simulink model "simulation_w_switch"  (Simulink 10.0)
settings: Solver=VariableStepAuto  StartTime=0.0  StopTime=tTot  MaxStep=1e-4  RelTol=1e-3
PreLoadFcn:
  | syst_init
values from neighbouring files (symbols this model uses):
  D = diag(Ir.^-1)    [syst_init.m]
  DGU = stateDyn(DGU,6)    [syst_init.m]
  Il_bar1 = 5/3    (= 1.66666666667)    [syst_init.m]
  Il_bar2 = 6/3    (= 2)    [syst_init.m]
  Il_bar3 = 7/3    (= 2.33333333333)    [syst_init.m]
  Il_bar4 = 6.5/3    (= 2.16666666667)    [syst_init.m]
  Il_bar5 = 8/3    (= 2.66666666667)    [syst_init.m]
  Il_bar6 = 7.5/3    (= 2.5)    [syst_init.m]
  L_first = Bc_first*Wcomm_first*(Bc_first')    [syst_init.m]
  L_full = Bc_full*Wcomm_full*(Bc_full')    [syst_init.m]
  L_unp = Bc_unp*Wcomm_unp*(Bc_unp')    [syst_init.m]
  N = 6    [syst_init.m]
  Pl_bar1 = 100/3    (= 33.3333333333)    [syst_init.m]
  Pl_bar2 = 120/3    (= 40)    [syst_init.m]
  Pl_bar3 = 105/3    (= 35)    [syst_init.m]
  Pl_bar4 = 95/3    (= 31.6666666667)    [syst_init.m]
  Pl_bar5 = 110/3    (= 36.6666666667)    [syst_init.m]
  Pl_bar6 = 105/3    (= 35)    [syst_init.m]
  T_zie_change = 17    [syst_init.m]
  T_zip_change = 6    [syst_init.m]
  Tc = 1.5    [syst_init.m]
  Tcommfail = tTot-3    (= 26)    [syst_init.m]
  Tplg = 10    [syst_init.m]
  Tunp = 22    [syst_init.m]
  Vref1 = 47    [syst_init.m]
  Vref2 = 48    [syst_init.m]
  Vref3 = 45    [syst_init.m]
  Vref4 = 50    [syst_init.m]
  Vref5 = 46    [syst_init.m]
  Vref6 = 49    [syst_init.m]
  Vs = 80    [syst_init.m]
  Yl_bar1 = 1/10/3    (= 0.0333333333333)    [syst_init.m]
  Yl_bar2 = 1/9/3    (= 0.037037037037)    [syst_init.m]
  Yl_bar3 = 1/11/3    (= 0.030303030303)    [syst_init.m]
  Yl_bar4 = 1/11/3    (= 0.030303030303)    [syst_init.m]
  Yl_bar5 = 1/10/3    (= 0.0333333333333)    [syst_init.m]
  Yl_bar6 = 1/10.5/3    (= 0.031746031746)    [syst_init.m]
undefined symbols (not defined in the file or in its folder): L
libraries: powerlib x135, powerlib_meascontrol x6
(part 2 of 2)

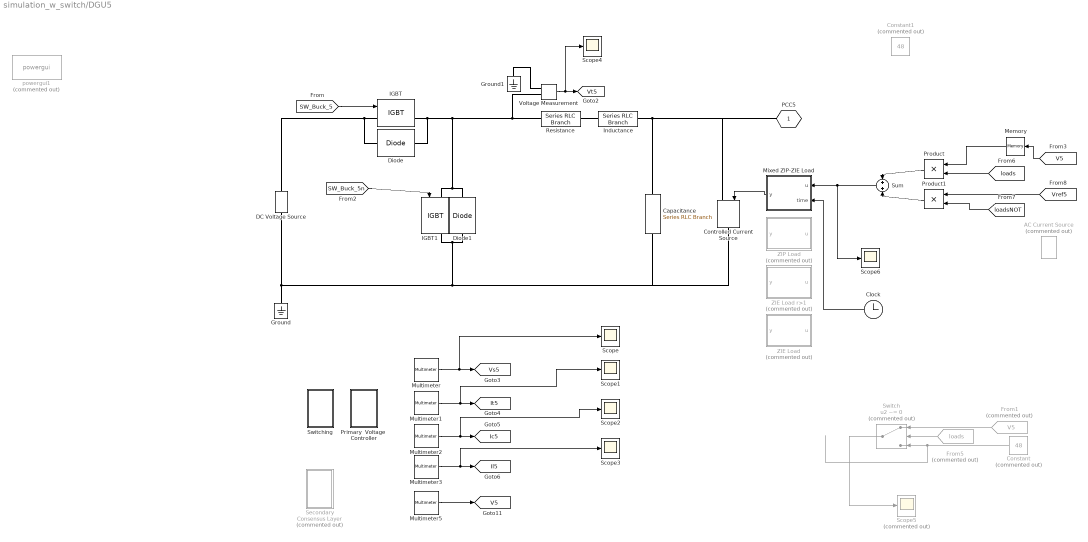
== system simulation_w_switch/DGU5 ==
  AC Current Source : powerlib/Electrical Sources/AC Current Source  Commented=on  Amplitude=18  Phase=90  Frequency=0  SampleTime=0  Measurements=Current
      settings: SourceProductName=Simscape Electrical  SourceProductBaseCode=PS
  Capacitance : powerlib/Elements/Series RLC Branch  LConnTagsString=__new0  RConnTagsString=__new0  BranchType=C  Resistance=1  Inductance=1.8e-3  SetiL0=off  InitialCurrent=0  Capacitance=DGU(5).Ct  Setx0=on  InitialVoltage=48  Measurements=Branch voltage and current
      settings: SourceProductName=Simscape Electrical
  Clock : Clock
  Constant : Constant  Commented=on  Value=48
  Constant1 : Constant  Commented=on  Value=48
  Controlled Current Source : powerlib/Electrical Sources/Controlled Current Source  Initialize=on  Source_Type=DC  Amplitude=Il_bar5  Phase=0  Frequency=0  Measurements=Current
      settings: SourceProductName=Simscape Electrical
  DC Voltage Source : powerlib/Electrical Sources/DC Voltage Source  Amplitude=Vs  Measurements=Voltage
      settings: SourceProductName=Simscape Electrical
  Diode : powerlib/Power Electronics/Diode  Ron=0.001  Lon=0  Vf=0.8  IC=0  UseSnubber=0  Rs=500  Cs=250e-9  Measurements=off
      settings: SourceProductName=Simscape Electrical
  Diode1 : powerlib/Power Electronics/Diode  Ron=0.001  Lon=0  Vf=0.8  IC=0  UseSnubber=0  Rs=500  Cs=250e-9  Measurements=off
      settings: SourceProductName=Simscape Electrical
  From1 : From  Commented=on  GotoTag=V5  TagVisibility=global
  From5 : From  Commented=on  GotoTag=loads  TagVisibility=global
  Ground : powerlib/Elements/Ground  LConnTagsString=a
      settings: SourceProductName=Simscape Electrical
  Ground1 : powerlib/Elements/Ground  LConnTagsString=a
      settings: SourceProductName=Simscape Electrical
  IGBT : powerlib/Power Electronics/IGBT  Ron=0.001  Lon=0  Vf=1  Tf=1e-6  Tt=2e-6  IC=0  Rs=1e5  Cs=inf  Measurements=on
      settings: SourceProductName=Simscape Electrical
  IGBT1 : powerlib/Power Electronics/IGBT  Ron=0.001  Lon=0  Vf=1  Tf=1e-6  Tt=2e-6  IC=0  Rs=1e5  Cs=inf  Measurements=on
      settings: SourceProductName=Simscape Electrical
  Inductance : powerlib/Elements/Series RLC Branch  LConnTagsString=__new0  RConnTagsString=__new0  BranchType=L  Resistance=1  Inductance=DGU(5).Lt  SetiL0=on  InitialCurrent=Il_bar5  Capacitance=1e-6  Setx0=off  InitialVoltage=0  Measurements=None
      settings: SourceProductName=Simscape Electrical
  Memory : Memory
  Mixed ZIP-ZIE Load : MATLAB Function  TreatAsAtomicUnit=on
  Multimeter : powerlib/Measurements/Multimeter  PhasorSimulation=off  OutputType=Complex  sel=11  L=30  Gain=1  yselected={'Usrc: DGU5/DC Voltage Source'};  PSBOutputType=1  PSBequivalent=0  AxesSetting=[0,0.1,-100,100]  Display=0  SavedBlockNames=-11
      settings: SourceProductName=Simscape Electrical
  Multimeter1 : powerlib/Measurements/Multimeter  PhasorSimulation=off  OutputType=Complex  sel=22  L=30  Gain=1  yselected={'Ib: DGU5/Resistance'};  PSBOutputType=1  PSBequivalent=0  AxesSetting=[0,0.1,-100,100]  Display=0  SavedBlockNames=-11
      settings: SourceProductName=Simscape Electrical
  Multimeter2 : powerlib/Measurements/Multimeter  PhasorSimulation=off  OutputType=Complex  sel=21  L=30  Gain=1  yselected={'Ib: DGU5/Capacitance'};  PSBOutputType=1  PSBequivalent=0  AxesSetting=[0,0.1,-100,100]  Display=0  SavedBlockNames=-11
      settings: SourceProductName=Simscape Electrical
  Multimeter3 : powerlib/Measurements/Multimeter  PhasorSimulation=off  OutputType=Complex  sel=29  L=30  Gain=1  yselected={'Isrc: DGU5/Controlled Current Source'};  PSBOutputType=1  PSBequivalent=0  AxesSetting=[0,0.1,-100,100]  Display=0  SavedBlockNames=-11
      settings: SourceProductName=Simscape Electrical
  Multimeter5 : powerlib/Measurements/Multimeter  PhasorSimulation=off  OutputType=Complex  sel=5  L=30  Gain=1  yselected={'Ub: DGU5/Capacitance'};  PSBOutputType=1  PSBequivalent=0  AxesSetting=[0,0.1,-100,100]  Display=0  SavedBlockNames=-11
      settings: SourceProductName=Simscape Electrical
  Primary  Voltage  Controller : Subsystem
  Product : Product
  Product1 : Product
  Resistance : powerlib/Elements/Series RLC Branch  LConnTagsString=__new0  RConnTagsString=__new0  BranchType=R  Resistance=DGU(5).Rt  Inductance=1e-3  SetiL0=off  InitialCurrent=0  Capacitance=1e-6  Setx0=off  InitialVoltage=0  Measurements=Branch current
      settings: SourceProductName=Simscape Electrical
  Scope{,1..4,6} (6 alike) : Scope
  Scope5 : Scope  Commented=on
  Secondary Consensus Layer : Subsystem  Commented=on
  Sum : Sum  Inputs=+|+
  Switch : Switch  Commented=on  Criteria=u2 ~= 0  Threshold=0.1  ZeroCross=off
  Switching : Subsystem
  Voltage Measurement : powerlib/Measurements/Voltage Measurement  PhasorSimulation=off  OutputType=Complex  PSBequivalent=0
      settings: SourceProductName=Simscape Electrical
  ZIE Load : MATLAB Function  Commented=on  TreatAsAtomicUnit=on
  ZIE Load r>1 : MATLAB Function  Commented=on  TreatAsAtomicUnit=on
  ZIP Load : MATLAB Function  Commented=on  TreatAsAtomicUnit=on
  powergui1 : powerlib/powergui  Priority=1  Commented=on  SimulationMode=Continuous  SampleTime=50e-6  frequency=60  Iterations=50  frequencyindice=60  Pbase=100e6  ErrMax=1e-4  UnitsV=kV  UnitsW=MW  buscounter=0  FunctionMessages=off  echomessages=off  EnableUseOfTLC=off  CurrentSourceSwitches=off  DisableSnubberDevices=off  DisableRonSwitches=off  DisableVfSwitches=off  DisplayEquations=off  AutomaticDiscreteSolvers=off  SolverType=Tustin/Backward Euler (TBE)  Interpol=off  ExternalGateDelay=off  methode=off  Ts=100  x0status=blocks  SPID=on  SwTol=0  HookPort=off  NonlinearTolerance=1e-4  nMaxIteration=100  ContinueOnMaxIteration=off  RestoreLinks=warning  ResistiveCurrentMeasurement=off  Frange=[0:2:500]  Ylog=off  Xlog=on  ShowGrid=off  save=off  variable=ZData  structure=0  ZoomFFT=off  StartTime=0.0  cycles=1  DisplayStyle=1  fundamental=60  FreqAxis=off  MaxFrequency=1000  frequencyindicesteady=1  RmsSteady=1  display=off
      settings: SourceProductName=Simscape Electrical
  PCC5 : PMIOPort  Tag=PMCPort  Side=Left
  tag scope: Ic5=global, Il5=global, It5=global, V5=global, Vs5=global, Vt5=global
  wires:
  Multimeter/1 -> Scope/1, [Vs5]
  Multimeter2/1 -> Scope2/1, [Ic5]
  Voltage Measurement/1 -> Scope4/1, [Vt5]
  Multimeter1/1 -> Scope1/1, [It5]
  [SW_Buck_5n] -> IGBT1/1
  Multimeter3/1 -> Scope3/1, [Il5]
  [SW_Buck_5] -> IGBT/1
  Multimeter5/1 -> [V5]
  Mixed ZIP-ZIE Load/1(y) -> Controlled Current Source/1
  From5/1 -> Switch/2
  From1/1 -> Switch/1
  Constant/1 -> Switch/3
  Switch/1 -> Scope5/1
  [Vref5] -> Product1/1
  Product1/1 -> Sum/2
  Sum/1 -> Mixed ZIP-ZIE Load/1(u), Scope6/1
  [loadsNOT] -> Product1/2
  [loads] -> Product/2
  Memory/1 -> Product/1
  Product/1 -> Sum/1
  [V5] -> Memory/1
  Clock/1 -> Mixed ZIP-ZIE Load/2(time)
  connections:
  Ground1/LConn1 -- Voltage Measurement/LConn2
  IGBT1/RConn1 -- Controlled Current Source/RConn1 -- Capacitance/RConn1 -- Ground/LConn1 -- DC Voltage Source/LConn1 -- Diode1/LConn1
  Capacitance/LConn1 -- Controlled Current Source/LConn1 -- PCC5/RConn1 -- Inductance/RConn1
  IGBT/LConn1 -- Diode/RConn1 -- DC Voltage Source/RConn1
  Resistance/RConn1 -- Inductance/LConn1
  IGBT/RConn1 -- Resistance/LConn1 -- Voltage Measurement/LConn1 -- Diode1/RConn1 -- IGBT1/LConn1 -- Diode/LConn1

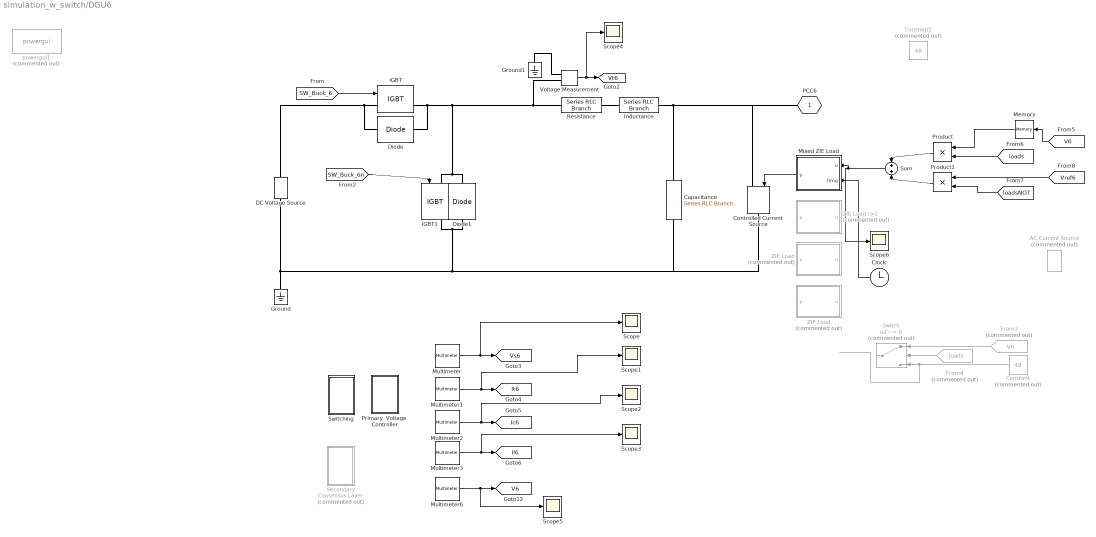
== system simulation_w_switch/DGU6 ==
  AC Current Source : powerlib/Electrical Sources/AC Current Source  Commented=on  Amplitude=16  Phase=90  Frequency=0  SampleTime=0  Measurements=Current
      settings: SourceProductName=Simscape Electrical  SourceProductBaseCode=PS
  Capacitance : powerlib/Elements/Series RLC Branch  LConnTagsString=__new0  RConnTagsString=__new0  BranchType=C  Resistance=1  Inductance=1.8e-3  SetiL0=off  InitialCurrent=0  Capacitance=DGU(6).Ct  Setx0=on  InitialVoltage=48  Measurements=Branch voltage and current
      settings: SourceProductName=Simscape Electrical
  Clock : Clock
  Constant : Constant  Commented=on  Value=48
  Constant1 : Constant  Commented=on  Value=48
  Controlled Current Source : powerlib/Electrical Sources/Controlled Current Source  Initialize=off  Source_Type=DC  Amplitude=Il_bar6  Phase=0  Frequency=0  Measurements=Current
      settings: SourceProductName=Simscape Electrical
  DC Voltage Source : powerlib/Electrical Sources/DC Voltage Source  Amplitude=Vs  Measurements=Voltage
      settings: SourceProductName=Simscape Electrical
  Diode : powerlib/Power Electronics/Diode  Ron=0.001  Lon=0  Vf=0.8  IC=0  UseSnubber=0  Rs=500  Cs=250e-9  Measurements=off
      settings: SourceProductName=Simscape Electrical
  Diode1 : powerlib/Power Electronics/Diode  Ron=0.001  Lon=0  Vf=0.8  IC=0  UseSnubber=0  Rs=500  Cs=250e-9  Measurements=off
      settings: SourceProductName=Simscape Electrical
  From3 : From  Commented=on  GotoTag=V6  TagVisibility=global
  From4 : From  Commented=on  GotoTag=loads  TagVisibility=global
  Ground : powerlib/Elements/Ground  LConnTagsString=a
      settings: SourceProductName=Simscape Electrical
  Ground1 : powerlib/Elements/Ground  LConnTagsString=a
      settings: SourceProductName=Simscape Electrical
  IGBT : powerlib/Power Electronics/IGBT  Ron=0.001  Lon=0  Vf=1  Tf=1e-6  Tt=2e-6  IC=0  Rs=1e5  Cs=inf  Measurements=on
      settings: SourceProductName=Simscape Electrical
  IGBT1 : powerlib/Power Electronics/IGBT  Ron=0.001  Lon=0  Vf=1  Tf=1e-6  Tt=2e-6  IC=0  Rs=1e5  Cs=inf  Measurements=on
      settings: SourceProductName=Simscape Electrical
  Inductance : powerlib/Elements/Series RLC Branch  LConnTagsString=__new0  RConnTagsString=__new0  BranchType=L  Resistance=1  Inductance=DGU(6).Lt  SetiL0=on  InitialCurrent=Il_bar6  Capacitance=1e-6  Setx0=off  InitialVoltage=0  Measurements=None
      settings: SourceProductName=Simscape Electrical
  Memory : Memory
  Mixed ZIE Load : MATLAB Function  TreatAsAtomicUnit=on
  Multimeter : powerlib/Measurements/Multimeter  PhasorSimulation=off  OutputType=Complex  sel=12  L=30  Gain=1  yselected={'Usrc: DGU6/DC Voltage Source'};  PSBOutputType=1  PSBequivalent=0  AxesSetting=[0,0.1,-100,100]  Display=0  SavedBlockNames=-11
      settings: SourceProductName=Simscape Electrical
  Multimeter1 : powerlib/Measurements/Multimeter  PhasorSimulation=off  OutputType=Complex  sel=24  L=30  Gain=1  yselected={'Ib: DGU6/Resistance'};  PSBOutputType=1  PSBequivalent=0  AxesSetting=[0,0.1,-100,100]  Display=0  SavedBlockNames=-11
      settings: SourceProductName=Simscape Electrical
  Multimeter2 : powerlib/Measurements/Multimeter  PhasorSimulation=off  OutputType=Complex  sel=23  L=30  Gain=1  yselected={'Ib: DGU6/Capacitance'};  PSBOutputType=1  PSBequivalent=0  AxesSetting=[0,0.1,-100,100]  Display=0  SavedBlockNames=-11
      settings: SourceProductName=Simscape Electrical
  Multimeter3 : powerlib/Measurements/Multimeter  PhasorSimulation=off  OutputType=Complex  sel=30  L=30  Gain=1  yselected={'Isrc: DGU6/Controlled Current Source'};  PSBOutputType=1  PSBequivalent=0  AxesSetting=[0,0.1,-100,100]  Display=0  SavedBlockNames=-11
      settings: SourceProductName=Simscape Electrical
  Multimeter6 : powerlib/Measurements/Multimeter  PhasorSimulation=off  OutputType=Complex  sel=6  L=30  Gain=1  yselected={'Ub: DGU6/Capacitance'};  PSBOutputType=1  PSBequivalent=0  AxesSetting=[0,0.1,-100,100]  Display=0  SavedBlockNames=-11
      settings: SourceProductName=Simscape Electrical
  Primary  Voltage  Controller : Subsystem
  Product : Product
  Product1 : Product
  Resistance : powerlib/Elements/Series RLC Branch  LConnTagsString=__new0  RConnTagsString=__new0  BranchType=R  Resistance=DGU(6).Rt  Inductance=1e-3  SetiL0=off  InitialCurrent=0  Capacitance=1e-6  Setx0=off  InitialVoltage=0  Measurements=Branch current
      settings: SourceProductName=Simscape Electrical
  Scope{,1..6} (7 alike) : Scope
  Secondary Consensus Layer : Subsystem  Commented=on
  Sum : Sum  Inputs=+|+
  Switch : Switch  Commented=on  Criteria=u2 ~= 0  Threshold=0.1
  Switching : Subsystem
  Voltage Measurement : powerlib/Measurements/Voltage Measurement  PhasorSimulation=off  OutputType=Complex  PSBequivalent=0
      settings: SourceProductName=Simscape Electrical
  ZIE Load : MATLAB Function  Commented=on  TreatAsAtomicUnit=on
  ZIE Load r>1 : MATLAB Function  Commented=on  TreatAsAtomicUnit=on
  ZIP Load : MATLAB Function  Commented=on  TreatAsAtomicUnit=on
  powergui1 : powerlib/powergui  Priority=1  Commented=on  SimulationMode=Continuous  SampleTime=50e-6  frequency=60  Iterations=50  frequencyindice=60  Pbase=100e6  ErrMax=1e-4  UnitsV=kV  UnitsW=MW  buscounter=0  FunctionMessages=off  echomessages=off  EnableUseOfTLC=off  CurrentSourceSwitches=off  DisableSnubberDevices=off  DisableRonSwitches=off  DisableVfSwitches=off  DisplayEquations=off  AutomaticDiscreteSolvers=off  SolverType=Tustin/Backward Euler (TBE)  Interpol=off  ExternalGateDelay=off  methode=off  Ts=100  x0status=blocks  SPID=on  SwTol=0  HookPort=off  NonlinearTolerance=1e-4  nMaxIteration=100  ContinueOnMaxIteration=off  RestoreLinks=warning  ResistiveCurrentMeasurement=off  Frange=[0:2:500]  Ylog=off  Xlog=on  ShowGrid=off  save=off  variable=ZData  structure=0  ZoomFFT=off  StartTime=0.0  cycles=1  DisplayStyle=1  fundamental=60  FreqAxis=off  MaxFrequency=1000  frequencyindicesteady=1  RmsSteady=1  display=off
      settings: SourceProductName=Simscape Electrical
  PCC6 : PMIOPort  Tag=PMCPort  Side=Right
  tag scope: Ic6=global, Il6=global, It6=global, V6=global, Vs6=global, Vt6=global
  wires:
  Multimeter/1 -> Scope/1, [Vs6]
  Multimeter2/1 -> Scope2/1, [Ic6]
  Voltage Measurement/1 -> Scope4/1, [Vt6]
  Multimeter1/1 -> Scope1/1, [It6]
  [SW_Buck_6n] -> IGBT1/1
  Multimeter3/1 -> Scope3/1, [Il6]
  [SW_Buck_6] -> IGBT/1
  Multimeter6/1 -> Scope5/1, [V6]
  Mixed ZIE Load/1(y) -> Controlled Current Source/1
  From3/1 -> Switch/1
  From4/1 -> Switch/2
  Constant/1 -> Switch/3
  [Vref6] -> Product1/1
  Product1/1 -> Sum/2
  Sum/1 -> Scope6/1, Mixed ZIE Load/1(u)
  [loadsNOT] -> Product1/2
  [loads] -> Product/2
  Memory/1 -> Product/1
  Product/1 -> Sum/1
  [V6] -> Memory/1
  Clock/1 -> Mixed ZIE Load/2(time)
  connections:
  Ground1/LConn1 -- Voltage Measurement/LConn2
  IGBT1/RConn1 -- Controlled Current Source/RConn1 -- Capacitance/RConn1 -- Ground/LConn1 -- DC Voltage Source/LConn1 -- Diode1/LConn1
  Capacitance/LConn1 -- Controlled Current Source/LConn1 -- PCC6/RConn1 -- Inductance/RConn1
  IGBT/LConn1 -- Diode/RConn1 -- DC Voltage Source/RConn1
  Resistance/RConn1 -- Inductance/LConn1
  IGBT/RConn1 -- Resistance/LConn1 -- Voltage Measurement/LConn1 -- Diode1/RConn1 -- IGBT1/LConn1 -- Diode/LConn1

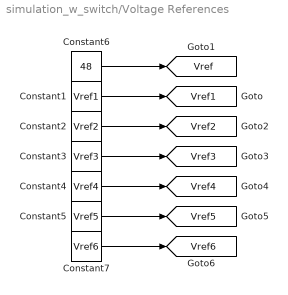
== system simulation_w_switch/Voltage References ==
  Constant1 : Constant  Value=Vref1
  Constant2 : Constant  Value=Vref2
  Constant3 : Constant  Value=Vref3
  Constant4 : Constant  Value=Vref4
  Constant5 : Constant  Value=Vref5
  Constant6 : Constant  Value=48
  Constant7 : Constant  Value=Vref6
  tag scope: Vref1=global, Vref2=global, Vref3=global, Vref4=global, Vref5=global, Vref6=global, Vref=global
  wires:
  Constant6/1 -> [Vref]
  Constant7/1 -> [Vref6]
  Constant5/1 -> [Vref5]
  Constant4/1 -> [Vref4]
  Constant3/1 -> [Vref3]
  Constant2/1 -> [Vref2]
  Constant1/1 -> [Vref1]

== system simulation_w_switch/DGU1/Primary  Voltage  Controller ==
  Gain1 : Gain  Gain=DGU(1).K  Multiplication=Matrix(K*u) (u vector)
  Integrator : Integrator
  Mux : Mux
  Sum : Sum  Inputs=-|+|-
  tag scope: Vt1d=global, x1=global
  wires:
  [It1] -> Mux/2
  Integrator/1 -> Mux/3
  Gain1/1 -> [Vt1d]
  Sum/1 -> Integrator/1
  Mux/1 -> [x1], Gain1/1
  [Vref1] -> Sum/2
  [V1] -> Mux/1, Sum/1
  [omega1] -> Mux/4, Sum/3

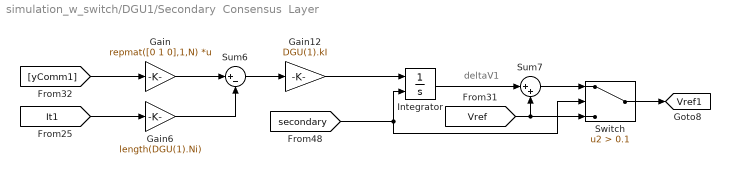
== system simulation_w_switch/DGU1/Secondary  Consensus  Layer ==
  note: deltaV1
  Gain : Gain  Gain=repmat([0 1 0],1,N)  Multiplication=Matrix(K*u) (u vector)
  Gain12 : Gain  Gain=DGU(1).kI
  Gain6 : Gain  Gain=length(DGU(1).Ni)
  Integrator : Integrator  ExternalReset=rising
  Sum6 : Sum  Inputs=|+-
  Sum7 : Sum  Inputs=|++
  Switch : Switch  Criteria=u2 > Threshold  Threshold=0.1
  tag scope: Vref1=global
  wires:
  [secondary] -> Integrator/2, Switch/2
  [yComm1] -> Gain/1
  Gain/1 -> Sum6/1
  Sum7/1 -> Switch/1
  Integrator/1 -> Sum7/1
  Switch/1 -> [Vref1]
  [Vref] -> Switch/3, Sum7/2
  [It1] -> Gain6/1
  Gain6/1 -> Sum6/2
  Sum6/1 -> Gain12/1
  Gain12/1 -> Integrator/1

== system simulation_w_switch/DGU1/Switching ==
  Divide : Product  Inputs=*/
  Logical Operator : Logic  Operator=NOT  AllPortsSameDT=off  OutDataTypeStr=boolean
  PWM Generator (DC-DC) : powerlib_meascontrol/Pulse & Signal Generators/PWM Generator (DC-DC)  Fsw=15000  Ts=0
      settings: SourceProductName=Simscape Electrical
  tag scope: SW_Buck_1=global, SW_Buck_1n=global, SW_Duty_1=global
  wires:
  [Vs1] -> Divide/2
  Logical Operator/1 -> [SW_Buck_1n]
  PWM Generator (DC-DC)/1 -> Logical Operator/1, [SW_Buck_1]
  Divide/1 -> [SW_Duty_1], PWM Generator (DC-DC)/1
  [Vt1d] -> Divide/1

== system simulation_w_switch/DGU2/Primary  Voltage  Controller ==
  Gain1 : Gain  Gain=DGU(2).K  Multiplication=Matrix(K*u) (u vector)
  Integrator : Integrator
  Mux : Mux
  Sum : Sum  Inputs=-|+|-
  tag scope: Vt2d=global, x2=global
  wires:
  [It2] -> Mux/2
  Integrator/1 -> Mux/3
  Gain1/1 -> [Vt2d]
  Sum/1 -> Integrator/1
  Mux/1 -> [x2], Gain1/1
  [Vref2] -> Sum/2
  [V2] -> Sum/1, Mux/1
  [omega2] -> Sum/3, Mux/4

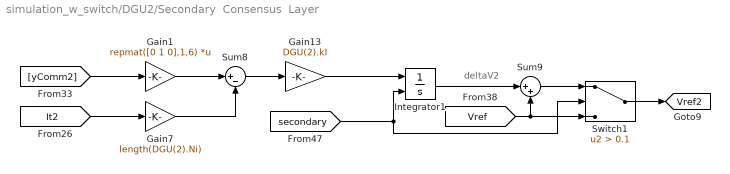
== system simulation_w_switch/DGU2/Secondary  Consensus  Layer ==
  note: deltaV2
  Gain1 : Gain  Gain=repmat([0 1 0],1,6)  Multiplication=Matrix(K*u) (u vector)
  Gain13 : Gain  Gain=DGU(2).kI
  Gain7 : Gain  Gain=length(DGU(2).Ni)
  Integrator1 : Integrator  ExternalReset=rising
  Sum8 : Sum  Inputs=|+-
  Sum9 : Sum  Inputs=|++
  Switch1 : Switch  Criteria=u2 > Threshold  Threshold=0.1
  tag scope: Vref2=global
  wires:
  [It2] -> Gain7/1
  Gain7/1 -> Sum8/2
  Gain1/1 -> Sum8/1
  [yComm2] -> Gain1/1
  Integrator1/1 -> Sum9/1
  Sum9/1 -> Switch1/1
  Sum8/1 -> Gain13/1
  [secondary] -> Integrator1/2, Switch1/2
  Switch1/1 -> [Vref2]
  Gain13/1 -> Integrator1/1
  [Vref] -> Switch1/3, Sum9/2

== system simulation_w_switch/DGU2/Switching ==
  Divide : Product  Inputs=*/
  Logical Operator : Logic  Operator=NOT  AllPortsSameDT=off  OutDataTypeStr=boolean
  PWM Generator (DC-DC) : powerlib_meascontrol/Pulse & Signal Generators/PWM Generator (DC-DC)  Fsw=15000  Ts=0
      settings: SourceProductName=Simscape Electrical
  tag scope: SW_Buck_2=global, SW_Buck_2n=global, SW_Duty_2=global
  wires:
  [Vs2] -> Divide/2
  Logical Operator/1 -> [SW_Buck_2n]
  PWM Generator (DC-DC)/1 -> Logical Operator/1, [SW_Buck_2]
  Divide/1 -> [SW_Duty_2], PWM Generator (DC-DC)/1
  [Vt2d] -> Divide/1

== system simulation_w_switch/DGU3/Primary  Voltage  Controller ==
  Gain1 : Gain  Gain=DGU(3).K  Multiplication=Matrix(K*u) (u vector)
  Integrator : Integrator
  Mux : Mux
  Sum : Sum  Inputs=-|+|-
  tag scope: Vt3d=global, x3=global
  wires:
  [It3] -> Mux/2
  Integrator/1 -> Mux/3
  Gain1/1 -> [Vt3d]
  Sum/1 -> Integrator/1
  Mux/1 -> [x3], Gain1/1
  [Vref3] -> Sum/2
  [V3] -> Mux/1, Sum/1
  [omega3] -> Sum/3, Mux/4

== system simulation_w_switch/DGU3/Secondary  Consensus Layer ==
  note: deltaV3
  Gain14 : Gain  Gain=DGU(3).kI
  Gain2 : Gain  Gain=repmat([0 1 0],1,6)  Multiplication=Matrix(K*u) (u vector)
  Gain8 : Gain  Gain=length(DGU(3).Ni)
  Integrator2 : Integrator  ExternalReset=rising
  Sum10 : Sum  Inputs=|+-
  Sum11 : Sum  Inputs=|++
  Switch2 : Switch  Criteria=u2 > Threshold  Threshold=0.1
  tag scope: Vref3=global
  wires:
  Gain8/1 -> Sum10/2
  [It3] -> Gain8/1
  Integrator2/1 -> Sum11/1
  [secondary] -> Integrator2/2, Switch2/2
  Gain2/1 -> Sum10/1
  [yComm3] -> Gain2/1
  Sum10/1 -> Gain14/1
  Gain14/1 -> Integrator2/1
  Switch2/1 -> [Vref3]
  Sum11/1 -> Switch2/1
  [Vref] -> Switch2/3, Sum11/2

== system simulation_w_switch/DGU3/Switching ==
  Divide : Product  Inputs=*/
  Logical Operator : Logic  Operator=NOT  AllPortsSameDT=off  OutDataTypeStr=boolean
  PWM Generator (DC-DC) : powerlib_meascontrol/Pulse & Signal Generators/PWM Generator (DC-DC)  Fsw=15000  Ts=0
      settings: SourceProductName=Simscape Electrical
  tag scope: SW_Buck_3=global, SW_Buck_3n=global, SW_Duty_3=global
  wires:
  [Vs3] -> Divide/2
  Logical Operator/1 -> [SW_Buck_3n]
  PWM Generator (DC-DC)/1 -> Logical Operator/1, [SW_Buck_3]
  Divide/1 -> [SW_Duty_3], PWM Generator (DC-DC)/1
  [Vt3d] -> Divide/1

== system simulation_w_switch/DGU4/Primary  Voltage  Controller ==
  Gain1 : Gain  Gain=DGU(4).K  Multiplication=Matrix(K*u) (u vector)
  Integrator : Integrator
  Mux : Mux
  Sum : Sum  Inputs=-|+|-
  tag scope: Vt4d=global, x4=global
  wires:
  [It4] -> Mux/2
  Integrator/1 -> Mux/3
  Gain1/1 -> [Vt4d]
  Sum/1 -> Integrator/1
  Mux/1 -> [x4], Gain1/1
  [Vref4] -> Sum/2
  [V4] -> Sum/1, Mux/1
  [omega4] -> Mux/4, Sum/3

== system simulation_w_switch/DGU4/Secondary Consensus Layer ==
  note: deltaV4
  Gain15 : Gain  Gain=DGU(4).kI
  Gain3 : Gain  Gain=repmat([0 1 0],1,6)  Multiplication=Matrix(K*u) (u vector)
  Gain9 : Gain  Gain=length(DGU(4).Ni)
  Integrator3 : Integrator  ExternalReset=rising
  Sum12 : Sum  Inputs=|+-
  Sum13 : Sum  Inputs=|++
  Switch3 : Switch  Criteria=u2 > Threshold  Threshold=0.1
  tag scope: Vref4=global
  wires:
  Gain3/1 -> Sum12/1
  Switch3/1 -> [Vref4]
  Integrator3/1 -> Sum13/1
  [It4] -> Gain9/1
  Sum12/1 -> Gain15/1
  Sum13/1 -> Switch3/1
  Gain15/1 -> Integrator3/1
  [secondary] -> Integrator3/2, Switch3/2
  [Vref] -> Switch3/3, Sum13/2
  [yComm4] -> Gain3/1
  Gain9/1 -> Sum12/2

== system simulation_w_switch/DGU4/Switching ==
  Divide : Product  Inputs=*/
  Logical Operator : Logic  Operator=NOT  AllPortsSameDT=off  OutDataTypeStr=boolean
  PWM Generator (DC-DC) : powerlib_meascontrol/Pulse & Signal Generators/PWM Generator (DC-DC)  Fsw=15000  Ts=0
      settings: SourceProductName=Simscape Electrical
  tag scope: SW_Buck_4=global, SW_Buck_4n=global, SW_Duty_4=global
  wires:
  [Vs4] -> Divide/2
  Logical Operator/1 -> [SW_Buck_4n]
  PWM Generator (DC-DC)/1 -> Logical Operator/1, [SW_Buck_4]
  Divide/1 -> [SW_Duty_4], PWM Generator (DC-DC)/1
  [Vt4d] -> Divide/1

== system simulation_w_switch/DGU5/Primary  Voltage  Controller ==
  Gain1 : Gain  Gain=DGU(5).K  Multiplication=Matrix(K*u) (u vector)
  Integrator : Integrator
  Mux : Mux
  Scope : Scope
  Sum : Sum  Inputs=-|+|-
  tag scope: Vt5d=global, x5=global
  wires:
  [It5] -> Mux/2
  Integrator/1 -> Mux/3
  Gain1/1 -> [Vt5d]
  Sum/1 -> Integrator/1
  Mux/1 -> Scope/1, [x5], Gain1/1
  [Vref5] -> Sum/2
  [V5] -> Mux/1, Sum/1
  [omega5] -> Mux/4, Sum/3

== system simulation_w_switch/DGU5/Secondary Consensus Layer ==
  note: deltaV5
  Gain10 : Gain  Gain=length(DGU(5).Ni)
  Gain16 : Gain  Gain=DGU(5).kI
  Gain4 : Gain  Gain=repmat([0 1 0],1,6)  Multiplication=Matrix(K*u) (u vector)
  Integrator4 : Integrator  ExternalReset=rising
  Sum14 : Sum  Inputs=|+-
  Sum15 : Sum  Inputs=|++
  Switch4 : Switch  Criteria=u2 > Threshold  Threshold=0.1
  tag scope: Vref5=global
  wires:
  Gain16/1 -> Integrator4/1
  Sum14/1 -> Gain16/1
  Gain4/1 -> Sum14/1
  Sum15/1 -> Switch4/1
  [It5] -> Gain10/1
  Integrator4/1 -> Sum15/1
  Switch4/1 -> [Vref5]
  [Vref] -> Switch4/3, Sum15/2
  [yComm5] -> Gain4/1
  Gain10/1 -> Sum14/2
  [secondary] -> Switch4/2, Integrator4/2

== system simulation_w_switch/DGU5/Switching ==
  Divide : Product  Inputs=*/
  Logical Operator : Logic  Operator=NOT  AllPortsSameDT=off  OutDataTypeStr=boolean
  PWM Generator (DC-DC) : powerlib_meascontrol/Pulse & Signal Generators/PWM Generator (DC-DC)  Fsw=15000  Ts=0
      settings: SourceProductName=Simscape Electrical
  tag scope: SW_Buck_5=global, SW_Buck_5n=global, SW_Duty_5=global
  wires:
  [Vs5] -> Divide/2
  Logical Operator/1 -> [SW_Buck_5n]
  PWM Generator (DC-DC)/1 -> Logical Operator/1, [SW_Buck_5]
  Divide/1 -> [SW_Duty_5], PWM Generator (DC-DC)/1
  [Vt5d] -> Divide/1

== system simulation_w_switch/DGU6/Primary  Voltage  Controller ==
  Gain1 : Gain  Gain=DGU(6).K  Multiplication=Matrix(K*u) (u vector)
  Integrator : Integrator
  Mux : Mux
  Scope : Scope
  Sum : Sum  Inputs=-|+|-
  tag scope: Vt6d=global, x6=global
  wires:
  [It6] -> Mux/2
  Integrator/1 -> Mux/3
  Gain1/1 -> [Vt6d]
  Sum/1 -> Integrator/1
  Mux/1 -> Scope/1, [x6], Gain1/1
  [Vref6] -> Sum/2
  [V6] -> Sum/1, Mux/1
  [omega6] -> Mux/4, Sum/3

== system simulation_w_switch/DGU6/Secondary Consensus Layer ==
  note: deltaV6
  Gain11 : Gain  Gain=length(DGU(6).Ni)
  Gain17 : Gain  Gain=DGU(6).kI
  Gain5 : Gain  Gain=repmat([0 1 0],1,6)  Multiplication=Matrix(K*u) (u vector)
  Integrator5 : Integrator  ExternalReset=rising
  Sum16 : Sum  Inputs=|+-
  Sum17 : Sum  Inputs=|++
  Switch5 : Switch  Criteria=u2 > Threshold  Threshold=0.1
  tag scope: Vref6=global
  wires:
  Switch5/1 -> [Vref6]
  Integrator5/1 -> Sum17/1
  Sum16/1 -> Gain17/1
  Gain11/1 -> Sum16/2
  [Vref] -> Switch5/3, Sum17/2
  Gain17/1 -> Integrator5/1
  Gain5/1 -> Sum16/1
  [secondary] -> Integrator5/2, Switch5/2
  [It6] -> Gain11/1
  Sum17/1 -> Switch5/1
  [yComm6] -> Gain5/1

== system simulation_w_switch/DGU6/Switching ==
  Divide : Product  Inputs=*/
  Logical Operator : Logic  Operator=NOT  AllPortsSameDT=off  OutDataTypeStr=boolean
  PWM Generator (DC-DC) : powerlib_meascontrol/Pulse & Signal Generators/PWM Generator (DC-DC)  Fsw=15000  Ts=0
      settings: SourceProductName=Simscape Electrical
  tag scope: SW_Buck_6=global, SW_Buck_6n=global, SW_Duty_6=global
  wires:
  [Vs6] -> Divide/2
  Logical Operator/1 -> [SW_Buck_6n]
  PWM Generator (DC-DC)/1 -> Logical Operator/1, [SW_Buck_6]
  Divide/1 -> [SW_Duty_6], PWM Generator (DC-DC)/1
  [Vt6d] -> Divide/1

== matlab function DGU3/ZIE Load r>1 ==
  data: u input double; y output double; Il_bar3 parameter double; Yl_bar3 parameter double; Pl_bar3 parameter double
function y = Il3(u, Il_bar3, Yl_bar3, Pl_bar3)

y = Il_bar3+Yl_bar3*u+Pl_bar3/30*(u^0.45);

== matlab function DGU1/ZIE Load ==
  data: u input double; y output double; Il_bar1 parameter double; Yl_bar1 parameter double; Pl_bar1 parameter double
function y = Il1(u, Il_bar1, Yl_bar1, Pl_bar1)

y = Il_bar1+Yl_bar1*u+Pl_bar1/(u^0.5);

== matlab function DGU3/ZIE Load ==
  data: u input double; y output double; Il_bar3 parameter double; Yl_bar3 parameter double; Pl_bar3 parameter double
function y = Il3(u, Il_bar3, Yl_bar3, Pl_bar3)

y = Il_bar3+Yl_bar3*u+Pl_bar3/(u^0.45);

== matlab function DGU1/ZIP Load ==
  data: u input double; y output double; Il_bar1 parameter double; Yl_bar1 parameter double; Pl_bar1 parameter double
function y = Il1(u, Il_bar1, Yl_bar1, Pl_bar1)

y = Il_bar1+Yl_bar1*u+Pl_bar1/(u^1);

== matlab function DGU4/ZIE Load ==
  data: u input double; y output double; Il_bar4 parameter double; Yl_bar4 parameter double; Pl_bar4 parameter double
function y = Il4(u, Il_bar4, Yl_bar4, Pl_bar4)

y = Il_bar4+Yl_bar4*u+Pl_bar4/(u^0.55);

== matlab function DGU2/ZIP Load ==
  data: u input double; y output double; Il_bar2 parameter double; Yl_bar2 parameter double; Pl_bar2 parameter double
function y = Il1(u, Il_bar2, Yl_bar2, Pl_bar2)

y = Il_bar2+Yl_bar2*u+Pl_bar2/(u^1);

== matlab function DGU6/ZIE Load ==
  data: u input double; y output double; Il_bar6 parameter double; Yl_bar6 parameter double; Pl_bar6 parameter double
function y = Il6(u, Il_bar6, Yl_bar6, Pl_bar6)

y = Il_bar6+Yl_bar6*u+Pl_bar6/(u^0.35);

== matlab function DGU3/ZIP Load ==
  data: u input double; y output double; Il_bar3 parameter double; Yl_bar3 parameter double; Pl_bar3 parameter double
function y = Il3(u, Il_bar3, Yl_bar3, Pl_bar3)

y = Il_bar3+Yl_bar3*u+Pl_bar3/(u^1);

== matlab function DGU5/ZIE Load ==
  data: u input double; y output double; Il_bar5 parameter double; Yl_bar5 parameter double; Pl_bar5 parameter double
function y = Il5(u, Il_bar5, Yl_bar5, Pl_bar5)

y = Il_bar5+Yl_bar5*u+Pl_bar5/(u^0.6);

== matlab function DGU4/ZIP Load ==
  data: u input double; y output double; Il_bar4 parameter double; Yl_bar4 parameter double; Pl_bar4 parameter double
function y = Il4(u, Il_bar4, Yl_bar4, Pl_bar4)

y = Il_bar4+Yl_bar4*u+Pl_bar4/(u^1);

== matlab function DGU5/ZIP Load ==
  data: u input double; y output double; Il_bar5 parameter double; Yl_bar5 parameter double; Pl_bar5 parameter double
function y = Il5(u, Il_bar5, Yl_bar5, Pl_bar5)

y = Il_bar5+Yl_bar5*u+Pl_bar5/(u^1);

== matlab function DGU6/ZIP Load ==
  data: u input double; y output double; Il_bar6 parameter double; Yl_bar6 parameter double; Pl_bar6 parameter double
function y = Il6(u, Il_bar6, Yl_bar6, Pl_bar6)

y = Il_bar6+Yl_bar6*u+Pl_bar6/(u^1);

== matlab function DGU1/ZIE Load r>1 ==
  data: u input double; y output double; Il_bar1 parameter double; Yl_bar1 parameter double; Pl_bar1 parameter double
function y = Il1(u, Il_bar1, Yl_bar1, Pl_bar1)

y = Il_bar1+Yl_bar1*u+Pl_bar1/50*(u^0.5);

== matlab function DGU2/ZIE Load r>1 ==
  data: u input double; y output double; Il_bar2 parameter double; Yl_bar2 parameter double; Pl_bar2 parameter double
function y = Il2(u, Il_bar2, Yl_bar2, Pl_bar2)

y = Il_bar2+Yl_bar2*u+Pl_bar2/50*(u^0.4);

== matlab function DGU4/ZIE Load r>1 ==
  data: u input double; y output double; Il_bar4 parameter double; Yl_bar4 parameter double; Pl_bar4 parameter double
function y = Il4(u, Il_bar4, Yl_bar4, Pl_bar4)

y = Il_bar4+Yl_bar4*u+Pl_bar4/50*(u^0.55);

== matlab function DGU5/ZIE Load r>1 ==
  data: u input double; y output double; Il_bar5 parameter double; Yl_bar5 parameter double; Pl_bar5 parameter double
function y = Il5(u, Il_bar5, Yl_bar5, Pl_bar5)

y = Il_bar5+Yl_bar5*u+Pl_bar5/30*(u^0.6);

== matlab function DGU6/ZIE Load r>1 ==
  data: u input double; y output double; Il_bar6 parameter double; Yl_bar6 parameter double; Pl_bar6 parameter double
function y = Il6(u, Il_bar6, Yl_bar6, Pl_bar6)

y = Il_bar6+Yl_bar6*u+Pl_bar6/50*(u^0.35);

== matlab function DGU2/ZIE Load ==
  data: u input double; y output double; Il_bar2 parameter double; Yl_bar2 parameter double; Pl_bar2 parameter double
function y = Il2(u, Il_bar2, Yl_bar2, Pl_bar2)

y = Il_bar2+Yl_bar2*u+Pl_bar2/(u^0.4);

== matlab function DGU6/Mixed ZIE Load ==
  data: u input double; time input double; y output double; Il_bar6 parameter double; Yl_bar6 parameter double; Pl_bar6 parameter double; T_zie_change parameter double
function y = Il6(u, time, Il_bar6, Yl_bar6, Pl_bar6, T_zie_change)

if time<T_zie_change
    y = Il_bar6+Yl_bar6*u+Pl_bar6/(u^0.35);
else
    y = Il_bar6+Yl_bar6*u+Pl_bar6/30*(u^0.35);
end

== matlab function DGU1/Mixed ZIP Load ==
  data: u input double; time input double; y output double; Il_bar1 parameter double; Yl_bar1 parameter double; Pl_bar1 parameter double; T_zip_change parameter double
function y = Il1(u, time, Il_bar1, Yl_bar1, Pl_bar1, T_zip_change)

if time<T_zip_change
    y = Il_bar1+Yl_bar1*u+Pl_bar1/(u^1);
else
    y = Il_bar1+1.3*Yl_bar1*u+1.3*Pl_bar1/(u^1);
end

== matlab function DGU4/Mixed ZIP Load ==
  data: u input double; time input double; y output double; Il_bar4 parameter double; Yl_bar4 parameter double; Pl_bar4 parameter double; T_zip_change parameter double
function y = Il4(u, time, Il_bar4, Yl_bar4, Pl_bar4, T_zip_change)

if time<T_zip_change
    y = Il_bar4+Yl_bar4*u+Pl_bar4/(u^1);
else
    y = Il_bar4+1.2*Yl_bar4*u+1.2*Pl_bar4/(u^1);
end

== matlab function DGU2/Mixed ZIP-ZIE Load ==
  data: u input double; time input double; y output double; Il_bar2 parameter double; Yl_bar2 parameter double; Pl_bar2 parameter double; Tplg parameter double
function y = Il2(u, time, Il_bar2, Yl_bar2, Pl_bar2, Tplg)

if time<Tplg
    y = Il_bar2+Yl_bar2*u+Pl_bar2/(u^1);
else
    y = Il_bar2+Yl_bar2*u+Pl_bar2/(u^0.4);
end

== matlab function DGU3/Mixed ZIP-ZIE Load ==
  data: u input double; time input double; y output double; Il_bar3 parameter double; Yl_bar3 parameter double; Pl_bar3 parameter double; Tplg parameter double; T_zie_change parameter double
function y = Il3(u, time, Il_bar3, Yl_bar3, Pl_bar3, Tplg, T_zie_change)

if time<Tplg
    y = Il_bar3+Yl_bar3*u+Pl_bar3/(u^1);
elseif time<T_zie_change
    y = Il_bar3+Yl_bar3*u+Pl_bar3/(u^0.45);
else
    y = Il_bar3+Yl_bar3*u+Pl_bar3/30*(u^0.45);
end

== matlab function DGU5/Mixed ZIP-ZIE Load ==
  data: u input double; time input double; y output double; Il_bar5 parameter double; Yl_bar5 parameter double; Pl_bar5 parameter double; Tplg parameter double
function y = Il5(u, time, Il_bar5, Yl_bar5, Pl_bar5, Tplg)

if time<Tplg
	y = Il_bar5+Yl_bar5*u+Pl_bar5/(u^1);
else
    y = Il_bar5+Yl_bar5*u+Pl_bar5/(u^0.6);
end
